simulink model "s_jsj4_7zhh_chqjzh001"  (Simulink 8.3)
settings: Solver=ode45  SolverMode=SingleTasking  StartTime=0.0  StopTime=1  FixedStep=0.1  RelTol=1e-3
settings Model: Creator=Zhu Supeng  LastModifiedBy=Zhu Supeng
settings DataIOCC: SignalLoggingName=sigsOut
settings DebuggingCC: SaveWithParameterizedLinksMsg=none  SignalResolutionControl=TryResolveAllWithWarning  SolverPrmCheckMsg=none  MultiTaskDSMMsg=warning  MultiTaskCondExecSysMsg=none  StateNameClashWarn=none
settings HardwareCC: TargetUnknown=on
settings RTWCC: IncludeERTFirstTime=on

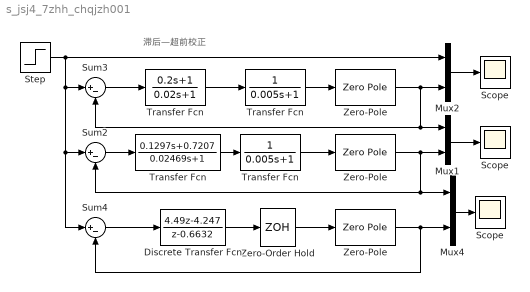
== system s_jsj4_7zhh_chqjzh001 ==
  note: 滞后—超前校正
  "  Transfer Fcn " : TransferFcn  Denominator=[0.005 1]
  "  Transfer Fcn   " : TransferFcn  Denominator=[0.005 1]
  " Discrete Transfer Fcn " : DiscreteTransferFcn  Numerator=[4.49 -4.247]  Denominator=[1 -0.6632]  SampleTime=0.01
  " Scope " : Scope
      settings: YMin=-3.5  YMax=1  SaveName=yyy  MaxDataPoints=500000
  " Zero-Pole " : ZeroPole  Zeros=[]  Poles=[0 -4]  Gain=[120]
  Mux1 : Mux  Inputs=2
  Mux2 : Mux  Inputs=2
  Mux4 : Mux  Inputs=2
  Scope : Scope
      settings: YMin=-3.5  YMax=1  MaxDataPoints=500000
  "Scope " : Scope
      settings: YMin=-3.5  YMax=1  SaveName=ScopeData2  MaxDataPoints=500000
  Step : Step  Time=0  SampleTime=0
  Sum2 : Sum  Inputs=|+-  SaturateOnIntegerOverflow=on
  Sum3 : Sum  Inputs=|+-  SaturateOnIntegerOverflow=on
  Sum4 : Sum  Inputs=|+-  SaturateOnIntegerOverflow=on
  Transfer Fcn : TransferFcn  Numerator=[0.2 1]  Denominator=[0.02 1]
  "Transfer Fcn " : TransferFcn  Numerator=[0.1297 0.7207]  Denominator=[0.02469 1]
  "Zero-Order Hold " : ZeroOrderHold  SampleTime=0.01
  Zero-Pole : ZeroPole  Zeros=[]  Poles=[0 -4]  Gain=[120]
  "Zero-Pole " : ZeroPole  Zeros=[]  Poles=[0 -4]  Gain=[120]
  wires:
  Step/1 -> Mux2/1, Sum3/1, Sum2/1, Sum4/1
  Mux2/1 -> "Scope "/1
  "Zero-Pole "/1 -> Mux2/2, Sum3/2, Mux1/1
  "  Transfer Fcn   "/1 -> "Zero-Pole "/1
  Mux4/1 -> " Scope "/1
  " Zero-Pole "/1 -> Mux4/2, Sum4/2
  " Discrete Transfer Fcn "/1 -> "Zero-Order Hold "/1
  Sum4/1 -> " Discrete Transfer Fcn "/1
  Mux1/1 -> Scope/1
  Zero-Pole/1 -> Mux1/2, Sum2/2, Mux4/1
  "Transfer Fcn "/1 -> "  Transfer Fcn "/1
  "  Transfer Fcn "/1 -> Zero-Pole/1
  Sum2/1 -> "Transfer Fcn "/1
  "Zero-Order Hold "/1 -> " Zero-Pole "/1
  Sum3/1 -> Transfer Fcn/1
  Transfer Fcn/1 -> "  Transfer Fcn   "/1
